simulink model "scout"  (R2018a)
settings: Solver=FixedStepAuto  StartTime=0.0  StopTime=20  FixedStep=0.01  RelTol=1e-3
undefined symbols (not defined in the file): sigbuilder_block
libraries: simulink x2
settings Model: EnablePacing=on  Creator=U500304  LastModifiedBy=U500304
settings SolverCC: ZeroCrossAlgorithm=Adaptive
settings DataIOCC: SaveOutput=off  SaveTime=off
settings DebuggingCC: MaxConsecutiveZCsMsg=none

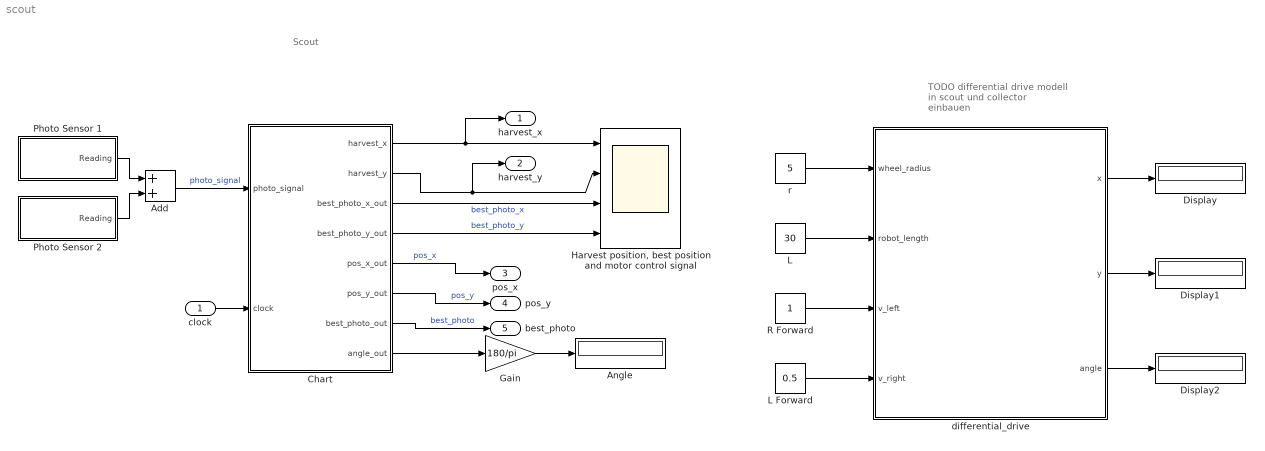
== system scout ==
  note: TODO differential drive
      | modell in scout und collector
      | einbauen
  note: Scout
  clock : Inport  OutDataTypeStr=double  PortDimensions=1  SampleTime=0
  Add : Sum
  Angle : Display
  Chart : Stateflow chart  TreatAsAtomicUnit=on
  Display : Display
  Display1 : Display
  Display2 : Display
  Gain : Gain  Gain=180/pi
  "Harvest position, best position and motor control signal" : Scope  NumInputPorts=4
  L : Constant  Value=30
  L Forward : Constant  Value=0.5
  Photo Sensor 1 : Subsystem  Tag=STV Subsys  LoadFcn=sigbuilder_block('load');  StartFcn=sigbuilder_block('start');  StopFcn=sigbuilder_block('stop');  ClipboardFcn=sigbuilder_block('clipboard');  mask(Sigbuilder block){tuvar=[0:10]}
      mask help: Simulink:masks:SigbuilderBlock_MD
      mask init:
      | if ~strcmp(get_param(bdroot(gcbh),'SimulationStatus'),'stopped') tuvar = sigbuilder_block('maskInit'); end
      settings: CopyFcn=sigbuilder_block('copy');  DeleteFcn=sigbuilder_block('delete');  ModelCloseFcn=sigbuilder_block('modelClose');  PreSaveFcn=sigbuilder_block('preSave');  PauseFcn=sigbuilder_block('pause');  ContinueFcn=sigbuilder_block('continue');  NameChangeFcn=sigbuilder_block('namechange');  OpenFcn=sigbuilder_block('open',[5.4 30 1141.2 522.6 ]);  CloseFcn=sigbuilder_block('close');
      mask Display: plot(0, 0, 100, 100,[2, 2, 32, 32, 2], [68, 8, 8, 68, 68],[32, 2], [38, 38], [32, 19, 2],[53, 60, 44], [32, 17, 17, 2],[16, 16, 31, 31]);txt = getActiveGroup(gcbh);text(2, 100, txt,'verticalAlignment', 'top');
  Photo Sensor 2 : Subsystem  Tag=STV Subsys  LoadFcn=sigbuilder_block('load');  StartFcn=sigbuilder_block('start');  StopFcn=sigbuilder_block('stop');  ClipboardFcn=sigbuilder_block('clipboard');  mask(Sigbuilder block){tuvar=[0:10]}
      mask help: Simulink:masks:SigbuilderBlock_MD
      mask init:
      | if ~strcmp(get_param(bdroot(gcbh),'SimulationStatus'),'stopped') tuvar = sigbuilder_block('maskInit'); end
      settings: CopyFcn=sigbuilder_block('copy');  DeleteFcn=sigbuilder_block('delete');  ModelCloseFcn=sigbuilder_block('modelClose');  PreSaveFcn=sigbuilder_block('preSave');  PauseFcn=sigbuilder_block('pause');  ContinueFcn=sigbuilder_block('continue');  NameChangeFcn=sigbuilder_block('namechange');  OpenFcn=sigbuilder_block('open',[5.4 30 1141.2 522.6 ]);  CloseFcn=sigbuilder_block('close');
      mask Display: plot(0, 0, 100, 100,[2, 2, 32, 32, 2], [68, 8, 8, 68, 68],[32, 2], [38, 38], [32, 19, 2],[53, 60, 44], [32, 17, 17, 2],[16, 16, 31, 31]);txt = getActiveGroup(gcbh);text(2, 100, txt,'verticalAlignment', 'top');
  R Forward : Constant
  differential_drive : Subsystem  TreatAsAtomicUnit=on
  r : Constant  Value=5
  harvest_x : Outport  OutDataTypeStr=double  PortDimensions=1  SampleTime=0
  harvest_y : Outport  Port=2  OutDataTypeStr=double  PortDimensions=1  SampleTime=0
  pos_x : Outport  Port=3  OutDataTypeStr=double  PortDimensions=1  SampleTime=0
  pos_y : Outport  Port=4  OutDataTypeStr=double  PortDimensions=1  SampleTime=0
  best_photo : Outport  Port=5  OutDataTypeStr=double  PortDimensions=1  SampleTime=0
  wires:
  Gain/1 -> Angle/1
  clock/1 -> Chart/2(clock)
  Add/1 -> Chart/1(photo_signal)  "photo_signal"
  Photo Sensor 2/1(Reading) -> Add/2
  Chart/6(pos_y_out) -> pos_y/1  "pos_y"
  Chart/4(best_photo_y_out) -> "Harvest position, best position and motor control signal"/4  "best_photo_y"
  Chart/8(angle_out) -> Gain/1
  Chart/3(best_photo_x_out) -> "Harvest position, best position and motor control signal"/3  "best_photo_x"
  Photo Sensor 1/1(Reading) -> Add/1
  Chart/1(harvest_x) -> "Harvest position, best position and motor control signal"/1, harvest_x/1
  Chart/2(harvest_y) -> harvest_y/1, "Harvest position, best position and motor control signal"/2
  Chart/5(pos_x_out) -> pos_x/1  "pos_x"
  Chart/7(best_photo_out) -> best_photo/1  "best_photo"
  r/1 -> differential_drive/1(wheel_radius)
  L/1 -> differential_drive/2(robot_length)
  R Forward/1 -> differential_drive/3(v_left)
  L Forward/1 -> differential_drive/4(v_right)
  differential_drive/1(x) -> Display/1
  differential_drive/2(y) -> Display1/1
  differential_drive/3(angle) -> Display2/1

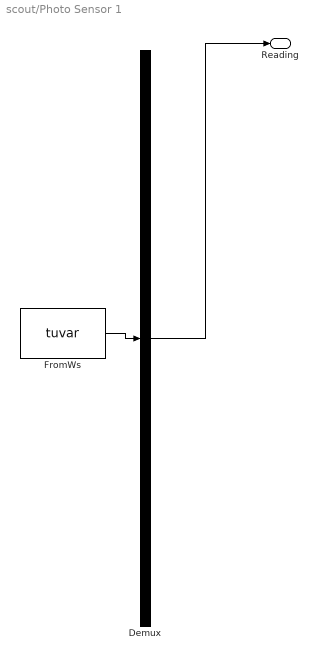
== system scout/Photo Sensor 1 ==
  Demux : Demux  Tag=STV Demux  Outputs=1
  FromWs : FromWorkspace  Tag=STV FromWs  VariableName=tuvar  SampleTime=0
      SigBuilderData=|
      | common.afterFinalStr = 'Extrapolate'
      | common.sampleTime = 0
      | dataSet.timeRange = [0 10]
      | dataSet.name = 'Photo Sensor'
      | sbobj.Groups.Name = 'Photo Sensor'
      | sbobj.Groups.Signals.Name = 'Reading'
      | sbobj.Groups.Signals.XData = [0 6 6 6.5 10]
      | sbobj.Groups.Signals.YData = [0 0 300 0 0]
  Reading : Outport  Tag=STV Outport
  wires:
  FromWs/1 -> Demux/1
  Demux/1 -> Reading/1

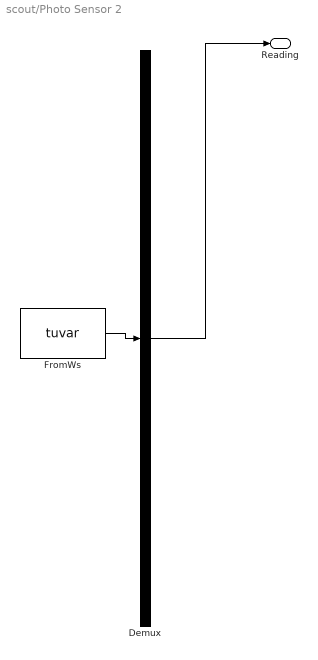
== system scout/Photo Sensor 2 ==
  Demux : Demux  Tag=STV Demux  Outputs=1
  FromWs : FromWorkspace  Tag=STV FromWs  VariableName=tuvar  SampleTime=0
      SigBuilderData=|
      | common.afterFinalStr = 'Extrapolate'
      | common.sampleTime = 0
      | dataSet.timeRange = [0 10]
      | dataSet.name = 'Photo Sensor'
      | sbobj.Groups.Name = 'Photo Sensor'
      | sbobj.Groups.Signals.Name = 'Reading'
      | sbobj.Groups.Signals.XData = [0 2 2 5 5 10]
      | sbobj.Groups.Signals.YData = [0 0 180 180 0 0]
  Reading : Outport  Tag=STV Outport
  wires:
  Demux/1 -> Reading/1
  FromWs/1 -> Demux/1

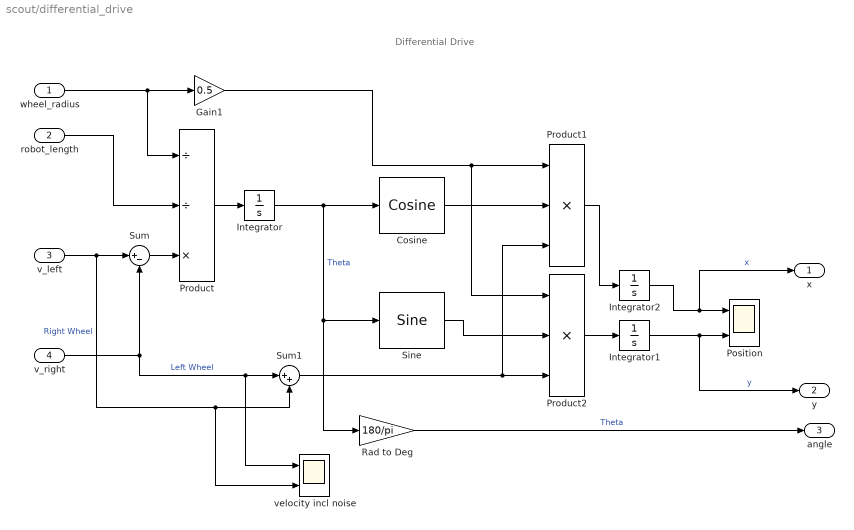
== system scout/differential_drive ==
  note: Differential Drive
  wheel_radius : Inport
  robot_length : Inport  Port=2
  v_left : Inport  Port=3
  v_right : Inport  Port=4
  Cosine : simulink/Lookup Tables/Cosine  Formula=cos(2*pi*u)  NumDataPoints=(2^5)+1  OutputWordLength=16  InternalRulePriority=Speed
      settings: SourceProductName=Simulink  SourceProductBaseCode=SL
  Gain1 : Gain  Gain=0.5
  Integrator : Integrator
  Integrator1 : Integrator
  Integrator2 : Integrator
  "Position " : Scope  NumInputPorts=2
  Product : Product  Inputs=//*
  Product1 : Product  Inputs=3
  Product2 : Product  Inputs=3
  Rad to Deg : Gain  Gain=180/pi
  Sine : simulink/Lookup Tables/Sine  Formula=sin(2*pi*u)  NumDataPoints=(2^5)+1  OutputWordLength=16  InternalRulePriority=Speed
      settings: SourceProductName=Simulink
  Sum : Sum  Inputs=|+-
  Sum1 : Sum  Inputs=|++
  velocity incl noise : Scope  NumInputPorts=2
  x : Outport
  y : Outport  Port=2
  angle : Outport  Port=3
  wires:
  Gain1/1 -> Product1/1, Product2/1
  Sum/1 -> Product/3
  Integrator/1 -> Rad to Deg/1, Sine/1, Cosine/1  "Theta"
  Integrator2/1 -> "Position "/1, x/1  "x"
  Cosine/1 -> Product1/2
  Sum1/1 -> Product1/3, Product2/3
  v_right/1 -> Sum/2, velocity incl noise/1, Sum1/1  "Left Wheel"
  robot_length/1 -> Product/2
  Sine/1 -> Product2/2
  Product/1 -> Integrator/1
  v_left/1 -> Sum/1, velocity incl noise/2, Sum1/2  "Right Wheel"
  Integrator1/1 -> "Position "/2, y/1  "y"
  Rad to Deg/1 -> angle/1  "Theta"
  Product2/1 -> Integrator1/1
  Product1/1 -> Integrator2/1
  wheel_radius/1 -> Product/1, Gain1/1

== stateflow chart scout/Chart ==
  settings: updateMethod=CONTINUOUS
  state Drive [parallel]
    settings: executionOrder=1
    state Move
      du:
      pos_x_dot = (r / 2) * (ul + ur) * cos(angle);
      pos_y_dot = (r / 2) * (ul + ur) * sin(angle);
      angle_dot = (r / L) * (ur - ul);
      pos_x_out = pos_x;
      pos_y_out = pos_y;
      angle_out = angle;
    note: Calculates robot's position based on wheel movements. Turns to 25 degrees left and drives straight on forever
    (default) -> Move : {
        | pos_x = 0;
        | pos_y = 0;
        | ul = 1;
        | ur = 1;
        | angle = 0;
        | turn = 0;
        | }
    Move -> Move [order 2] : [false]
        | {ul = 1; ur = -1; turn == 2;}
    Move -> Move [order 1] : [angle * 180/pi == 0 && turn == 0]
        | {ul = -1; ur = 1; turn = 1;}
    Move -> Move [order 3] : [angle * 180/pi  >= 25 && turn > 0]
        | {ul = 1; ur = 1; turn = 0}
  state Sense [parallel]
    settings: executionOrder=2
    state Dark
    state Light
      en, du:
      harvest_x = pos_x;
      harvest_y = pos_y;
    note: Senses the light and outputs harvest positions
    (default) -> Dark : {
        | best_photo = -1;
        | best_photo_x = -1;
        | best_photo_y = -1;
        | }
    Dark -> Light [order 1] : [photo_signal > 200]
    Dark -> Dark [order 2] : [photo_signal > best_photo]
        | {best_photo = photo_signal;
        | best_photo_x = pos_x;
        | best_photo_y = pos_y;}
    Light -> Dark [order 2] : [photo_signal <= 200]
    Light -> Light [order 1] : [photo_signal > best_photo]
        | {best_photo = photo_signal;
        | best_photo_x = pos_x;
        | best_photo_y = pos_y;}
  state Clock [parallel]
    settings: executionOrder=3
    state Seeking
      en:
      cycle_start = clock;
    state Report
      en:
      best_photo_out = best_photo;
      best_photo_x_out = best_photo_x;
      best_photo_y_out = best_photo_y;
    note: Updates the best harvest position
        | and light reading every 2 seconds
    (default) -> Seeking
    Report -> Seeking
    Seeking -> Report : [clock - cycle_start >= 2]
  data: photo_signal input; harvest_x output =-1; harvest_y output =-1; best_photo_x_out output =-1; best_photo_y_out output =-1; pos_x_out output; pos_y_out output; pos_x local; pos_y local; clock input; best_photo_out output =-1; best_photo local =0; best_photo_x local; best_photo_y local; cycle_start local; ur local double =1; ul local =1; angle local =0; r constant double =10; L constant double =100; angle_out output; turn local
  data pos_x settings: updateMethod=SF_CONTINUOUS_TIME_DATA
  data pos_y settings: updateMethod=SF_CONTINUOUS_TIME_DATA
  data angle settings: updateMethod=SF_CONTINUOUS_TIME_DATA
